simulink model "Demo_FrictionSensor_cs"  (Simulink 7.6)
settings: Solver=ode5  SolverMode=SingleTasking  StartTime=0.0  StopTime=12  FixedStep=1/200  RelTol=1e-3
PreLoadFcn:
  | check_NUTS_defined;
  | 
  | assignin('base',['model_closed_' bdroot],false);
InitFcn:
  | PreScanExperimentInitFcn(bdroot)
StopFcn:
  | PreScanExperimentStopFcn(bdroot)
undefined symbols (not defined in the file): DiscIntNeverNeededParam, warningInitialVelocity, x0, x_ini_VRML, y_ini_VRML, z_ini_VRML
libraries: simulink x40, PreScanSimulinkLibrary x15, simulink_extras x9, PreScanUsefulBlocks x3
(part 4 of 7)

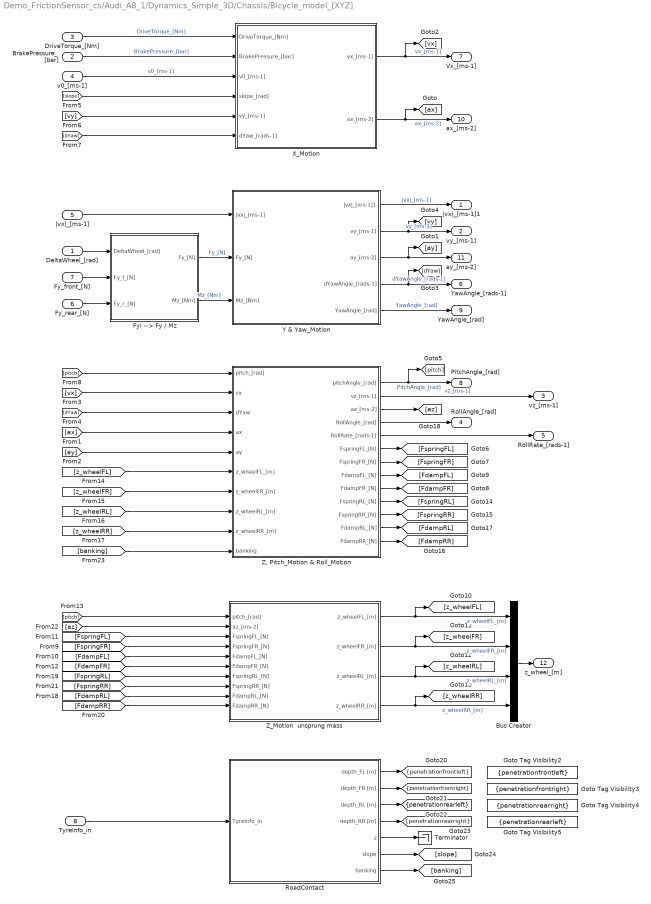
== system Demo_FrictionSensor_cs/Audi_A8_1/Dynamics_Simple_3D/Chassis/Bicycle_model_[XYZ] ==
  DeltaWheel_[rad] : Inport
  BrakePressure_[bar] : Inport  Port=2
  DriveTorque_[Nm] : Inport  Port=3
  v0_[ms-1] : Inport  Port=4
  |vx|_[ms-1] : Inport  Port=5
  Fy_rear_[N] : Inport  Port=6
  Fy_front_[N] : Inport  Port=7
  TyreInfo_in : Inport  Port=8
  Bus Creator : BusCreator
  Fyi --> Fy / Mz : Subsystem
  Goto Tag Visibility2 : GotoTagVisibility  GotoTag=penetrationfrontleft
  Goto Tag Visibility3 : GotoTagVisibility  GotoTag=penetrationfrontright
  Goto Tag Visibility4 : GotoTagVisibility  GotoTag=penetrationrearright
  Goto Tag Visibility5 : GotoTagVisibility  GotoTag=penetrationrearleft
  RoadContact : Subsystem
  Terminator : Terminator
  X_Motion : Subsystem
  Y & Yaw_Motion : Subsystem
  "Z, Pitch_Motion & Roll_Motion" : Subsystem
  Z_Motion  unsprung mass : Subsystem
  |vx|_[ms-1]1 : Outport
  vy_[ms-1] : Outport  Port=2
  vz_[ms-1] : Outport  Port=3
  RollAngle_[rad] : Outport  Port=4
  RollRate_[rads-1] : Outport  Port=5
  YawAngle_[rads-1] : Outport  Port=6
  Vx_[ms-1] : Outport  Port=7
  PitchAngle_[rad] : Outport  Port=8
  YawAngle_[rad] : Outport  Port=9
  ax_[ms-2] : Outport  Port=10
  ay_[ms-2] : Outport  Port=11
  z_wheel_[m] : Outport  Port=12
  tag scope: penetrationfrontleft=scoped, penetrationfrontright=scoped, penetrationrearleft=scoped, penetrationrearright=scoped
  wires:
  [banking] -> "Z, Pitch_Motion & Roll_Motion"/10(banking)
  RoadContact/7(banking) -> [banking]
  RoadContact/6(slope) -> [slope]
  RoadContact/5(z) -> Terminator/1
  "Z, Pitch_Motion & Roll_Motion"/1(pitchAngle_[rad]) -> PitchAngle_[rad]/1, [pitch]  "PitchAngle_[rad]"
  Y & Yaw_Motion/4(dYawAngle_[rads-1]) -> [dYaw], YawAngle_[rads-1]/1  "dYawAngle_[rads-1]"
  [vx] -> "Z, Pitch_Motion & Roll_Motion"/2(vx)
  [dYaw] -> "Z, Pitch_Motion & Roll_Motion"/3(dYaw)
  "Z, Pitch_Motion & Roll_Motion"/4(RollAngle_[rad]) -> RollAngle_[rad]/1
  [ay] -> "Z, Pitch_Motion & Roll_Motion"/5(ay)
  Y & Yaw_Motion/3(ay_[ms-2]) -> ay_[ms-2]/1, [ay]
  |vx|_[ms-1]/1 -> Y & Yaw_Motion/1(|vx|_[ms-1])
  Fy_rear_[N]/1 -> Fyi --> Fy / Mz/3(Fy_r_[N])
  Fy_front_[N]/1 -> Fyi --> Fy / Mz/2(Fy_f_[N])
  DeltaWheel_[rad]/1 -> Fyi --> Fy / Mz/1(DeltaWheel_[rad])
  [ax] -> "Z, Pitch_Motion & Roll_Motion"/4(ax)
  X_Motion/1(vx_[ms-1]) -> [vx], Vx_[ms-1]/1  "vx_[ms-1]"
  X_Motion/2(ax_[ms-2]) -> [ax], ax_[ms-2]/1  "ax_[ms-2]"
  DriveTorque_[Nm]/1 -> X_Motion/1(DriveTorque_[Nm])  "DriveTorque_[Nm]"
  BrakePressure_[bar]/1 -> X_Motion/2(BrakePressure_[bar])  "BrakePressure_[bar]"
  Y & Yaw_Motion/2(vy_[ms-1]) -> vy_[ms-1]/1, [vy]  "vy_[ms-1]"
  Y & Yaw_Motion/1(|vx|_[ms-1]1) -> |vx|_[ms-1]1/1  "|vx|_[ms-1]"
  Fyi --> Fy / Mz/2(Mz_[Nm]) -> Y & Yaw_Motion/3(Mz_[Nm])  "Mz_[Nm]"
  Fyi --> Fy / Mz/1(Fy_[N]) -> Y & Yaw_Motion/2(Fy_[N])  "Fy_[N]"
  [vy] -> X_Motion/5(vy_[ms-1])
  [dYaw] -> X_Motion/6(dYaw_[rads-1])
  "Z, Pitch_Motion & Roll_Motion"/3(az_[ms-2]) -> [az]
  "Z, Pitch_Motion & Roll_Motion"/5(RollRate_[rads-1]) -> RollRate_[rads-1]/1
  "Z, Pitch_Motion & Roll_Motion"/6(FspringFL_[N]) -> [FspringFL]
  "Z, Pitch_Motion & Roll_Motion"/7(FspringFR_[N]) -> [FspringFR]
  "Z, Pitch_Motion & Roll_Motion"/8(FdampFL_[N]) -> [FdampFL]
  "Z, Pitch_Motion & Roll_Motion"/9(FdampFR_[N]) -> [FdampFR]
  "Z, Pitch_Motion & Roll_Motion"/10(FspringRL_[N]) -> [FspringRL]
  "Z, Pitch_Motion & Roll_Motion"/11(FspringRR_[N]) -> [FspringRR]
  "Z, Pitch_Motion & Roll_Motion"/12(FdampRL_[N]) -> [FdampRL]
  "Z, Pitch_Motion & Roll_Motion"/13(FdampRR_[N]) -> [FdampRR]
  [pitch] -> "Z, Pitch_Motion & Roll_Motion"/1(pitch_[rad])
  [z_wheelFL] -> "Z, Pitch_Motion & Roll_Motion"/6(z_wheelFL_[m])
  [z_wheelFR] -> "Z, Pitch_Motion & Roll_Motion"/7(z_wheelFR_[m])
  [z_wheelRL] -> "Z, Pitch_Motion & Roll_Motion"/8(z_wheelRL_[m])
  [z_wheelRR] -> "Z, Pitch_Motion & Roll_Motion"/9(z_wheelRR_[m])
  Z_Motion  unsprung mass/1(z_wheelFL_[m]) -> [z_wheelFL], Bus Creator/1  "z_wheelFL_[m]"
  Z_Motion  unsprung mass/2(z_wheelFR_[m]) -> [z_wheelFR], Bus Creator/2  "z_wheelFR_[m]"
  Z_Motion  unsprung mass/3(z_wheelRL_[m]) -> [z_wheelRL], Bus Creator/3  "z_wheelRL_[m]"
  Z_Motion  unsprung mass/4(z_wheelRR_[m]) -> [z_wheelRR], Bus Creator/4  "z_wheelRR_[m]"
  [pitch] -> Z_Motion  unsprung mass/1(pitch_[rad])
  [FspringFL] -> Z_Motion  unsprung mass/3(FspringFL_[N])
  [FspringFR] -> Z_Motion  unsprung mass/4(FspringFR_[N])
  [FdampFL] -> Z_Motion  unsprung mass/5(FdampFL_[N])
  [FdampFR] -> Z_Motion  unsprung mass/6(FdampFR_[N])
  [FspringRL] -> Z_Motion  unsprung mass/7(FspringRL_[N])
  [FspringRR] -> Z_Motion  unsprung mass/8(FspringRR_[N])
  [FdampRL] -> Z_Motion  unsprung mass/9(FdampRL_[N])
  [FdampRR] -> Z_Motion  unsprung mass/10(FdampRR_[N])
  [az] -> Z_Motion  unsprung mass/2(az_[ms-2])
  Y & Yaw_Motion/5(YawAngle_[rad]) -> YawAngle_[rad]/1  "YawAngle_[rad]"
  RoadContact/1(depth_FL [m]) -> [penetrationfrontleft]
  RoadContact/2(depth_FR [m]) -> [penetrationfrontright]
  RoadContact/3(depth_RL [m]) -> [penetrationrearleft]
  RoadContact/4(depth_RR [m]) -> [penetrationrearright]
  [slope] -> X_Motion/4(slope_[rad])
  v0_[ms-1]/1 -> X_Motion/3(v0_[ms-1])  "v0_[ms-1]"
  "Z, Pitch_Motion & Roll_Motion"/2(vz_[ms-1]) -> vz_[ms-1]/1  "vz_[ms-1]"
  Bus Creator/1 -> z_wheel_[m]/1
  TyreInfo_in/1 -> RoadContact/1(TyreInfo_in)

== system Demo_FrictionSensor_cs/Audi_A8_1/Dynamics_Simple_3D/Chassis/FrontTyre ==
  note: alpha limiter
      | [-1 ... 1]
  note: VEHICLE + MOTORCYCLE
  note: MOTORCYCLE ONLY
  note: relax_on
      | ON: 1
      | OFF: 0
  DeltaWheel_[rad] : Inport
  |vx|_[ms-1] : Inport  Port=2
  vy_[ms-1] : Inport  Port=3
  dYawAngle_[rads-1] : Inport  Port=4
  RollAngle_[rad] : Inport  Port=5
  AlphaFront : Subsystem
  Compare To Zero : simulink/Logic and Bit Operations/Compare To Zero  SystemSampleTime=-1  relop===  LogicOutDataTypeMode=boolean  ZeroCross=off
  Configurable Subsystem : Subsystem  BlockChoice=Discrete-Time Integrator  mask{ComputationMode=ComputationMode}
      mask prompts: ComputationMode "Computation mode:"
      mask init:
      | SetComputationMode(gcb,ComputationMode);
      settings: AttributesFormatString=%<BlockChoice>  OpenFcn=BringToFront(gcb);  MemberBlocks=Discrete-Time Integrator,Integrator
      settings: TemplateBlock=|
      | PreScanSimulinkLibrary/Configurable Subsystems/integral with reset and limits
      | for slip angle/Configurable
      | Subsystem
  Configurable Subsystem1 : Subsystem  BlockChoice=Discrete-Time Integrator  mask{ComputationMode=ComputationMode}
      mask prompts: ComputationMode "Computation mode:"
      mask init:
      | SetComputationMode(gcb,ComputationMode);
      settings: AttributesFormatString=%<BlockChoice>  OpenFcn=BringToFront(gcb);  MemberBlocks=Discrete-Time Integrator,Integrator
      settings: TemplateBlock=|
      | PreScanSimulinkLibrary/Configurable Subsystems/integral with reset/Configurable
      | Subsystem
  Constant : Constant  Value=p.relax_on
  Constant1 : Constant  Value=p.relax_on
  Constant2 : Constant  Value=p.VehMCSwitch
  Data Type Conversion : DataTypeConversion  OutDataTypeStr=double
  If MC : simulink/Logic and Bit Operations/Compare To Constant  SystemSampleTime=-1  relop===  const=2  LogicOutDataTypeMode=uint8  ZeroCross=off
  K_gamma_front : Gain  Gain=p.Kgfront
  Linl : Fcn  Expr=(u(4) - u(5))/p.sigma_front*u(1)
  Linl1 : Fcn  Expr=(u(4) - u(5))/p.sigma_front*u(1)
  Mux1 : Mux  Inputs=3
  Mux2 : Mux  Inputs={3,1,1}
  Mux3 : Mux  Inputs={3,1,1}
  Product : Product  RndMeth=Zero
  Sum : Sum  Inputs=|++  SaturateOnIntegerOverflow=on  InputSameDT=on  OutDataTypeStr=Inherit: Same as first input
  Sum1 : Sum  Inputs=|++
  Switch : Switch  Threshold=0.5  SaturateOnIntegerOverflow=on  InputSameDT=on
  Switch1 : Switch  Threshold=0.5  SaturateOnIntegerOverflow=on  InputSameDT=on
  alg.loop : Memory
  due to sign convention : Gain  Gain=-1  SaturateOnIntegerOverflow=on  OutDataTypeStr=Inherit: Same as input  ParamDataTypeStr=Inherit: Same as input
  front_tyre : Gain  Gain=p.Kfront
  FyFront_[N] : Outport
  wires:
  Switch1/1 -> K_gamma_front/1  "GammaFront_[rad]"
  DeltaWheel_[rad]/1 -> Sum/2  "DeltaWheel_[rad]"
  [reset] -> Configurable Subsystem1/2(In2)
  [reset] -> Configurable Subsystem/2(In2)
  Compare To Zero/1 -> [reset]
  Data Type Conversion/1 -> Product/2
  Product/1 -> Sum1/2
  K_gamma_front/1 -> Product/1
  If MC/1 -> Data Type Conversion/1
  Constant2/1 -> If MC/1
  front_tyre/1 -> Sum1/1
  RollAngle_[rad]/1 -> due to sign convention/1
  due to sign convention/1 -> Mux3/2, alg.loop/1  "GammaStatFront_[rad]"
  Constant1/1 -> Switch1/2
  Mux3/1 -> Linl1/1
  Linl1/1 -> Configurable Subsystem1/1(In1)
  Configurable Subsystem1/1(Out1) -> Switch1/1, Mux3/3  "GammaRelaxFront_[rad]"
  alg.loop/1 -> Switch1/3
  dYawAngle_[rads-1]/1 -> Mux1/3
  vy_[ms-1]/1 -> Mux1/2
  |vx|_[ms-1]/1 -> Compare To Zero/1, Mux1/1
  Mux1/1 -> Mux3/1, Mux2/1, AlphaFront/1(In)
  AlphaFront/1(Alpha) -> Sum/1
  Configurable Subsystem/1(Out1) -> Switch/1, Mux2/3  "AlphaRelaxFront_[rad]"
  Linl/1 -> Configurable Subsystem/1(In1)
  Mux2/1 -> Linl/1
  Sum1/1 -> FyFront_[N]/1  "FyFront_[N]"
  Constant/1 -> Switch/2
  Switch/1 -> front_tyre/1  "AlphaFront_[rad]"
  Sum/1 -> Switch/3, Mux2/2  "AlphaStatFront_[rad]"

== system Demo_FrictionSensor_cs/Audi_A8_1/Dynamics_Simple_3D/Chassis/Power Assisted Steering ==
  note: Reverse steering direction for negative velocities
  note: VEHICLE
  note: MOTORCYCLE
  Vx_[ms-1] : Inport
  Delta_in_[deg] : Inport  Port=2
  Constant : Constant
  Constant1 : Constant  Value=p.VehMCSwitch
  Lookup Table : Lookup  InputValues=[0 35 45 100]  Table=[1 1 0.2 0.2]
  Multiport Switch : MultiPortSwitch  Inputs=2  zeroidx=off
  Product : Product  Inputs=3  RndMeth=Zero
  Sign : Signum
  Delta_out_[deg] : Outport
  wires:
  Sign/1 -> Product/1
  Product/1 -> Delta_out_[deg]/1
  Multiport Switch/1 -> Product/2
  Lookup Table/1 -> Multiport Switch/2
  Constant/1 -> Multiport Switch/3
  Constant1/1 -> Multiport Switch/1
  Delta_in_[deg]/1 -> Product/3
  Vx_[ms-1]/1 -> Sign/1, Lookup Table/1

== system Demo_FrictionSensor_cs/Audi_A8_1/Dynamics_Simple_3D/Chassis/RearTyre ==
  note: alpha limiter
      | [-1 ... 1]
  note: VEHICLE + MOTORCYCLE
  note: MOTORCYCLE ONLY
  note: relax_on
      | ON: 1
      | OFF: 0
  |vx|_[ms-1] : Inport
  vy_[ms-1] : Inport  Port=2
  dpsi_[rads-1] : Inport  Port=3
  RollAngle_[rad] : Inport  Port=4
  AlphaRear : Subsystem
  Compare To Zero : simulink/Logic and Bit Operations/Compare To Zero  SystemSampleTime=-1  relop===  LogicOutDataTypeMode=boolean  ZeroCross=off
  Configurable Subsystem : Subsystem  BlockChoice=Discrete-Time Integrator  mask{ComputationMode=ComputationMode}
      mask prompts: ComputationMode "Computation mode:"
      mask init:
      | SetComputationMode(gcb,ComputationMode);
      settings: AttributesFormatString=%<BlockChoice>  OpenFcn=BringToFront(gcb);  MemberBlocks=Discrete-Time Integrator,Integrator
      settings: TemplateBlock=|
      | PreScanSimulinkLibrary/Configurable Subsystems/integral with reset and limits
      | for slip angle/Configurable
      | Subsystem
  Configurable Subsystem1 : Subsystem  BlockChoice=Discrete-Time Integrator  mask{ComputationMode=ComputationMode}
      mask prompts: ComputationMode "Computation mode:"
      mask init:
      | SetComputationMode(gcb,ComputationMode);
      settings: AttributesFormatString=%<BlockChoice>  OpenFcn=BringToFront(gcb);  MemberBlocks=Discrete-Time Integrator,Integrator
      settings: TemplateBlock=|
      | PreScanSimulinkLibrary/Configurable Subsystems/integral with reset/Configurable
      | Subsystem
  Constant1 : Constant  Value=p.relax_on
  Constant2 : Constant  Value=p.relax_on
  Constant3 : Constant  Value=p.VehMCSwitch
  Data Type Conversion : DataTypeConversion  OutDataTypeStr=double
  If MC : simulink/Logic and Bit Operations/Compare To Constant  SystemSampleTime=-1  relop===  const=2  LogicOutDataTypeMode=uint8  ZeroCross=off
  K_gamma_rear : Gain  Gain=p.Kgrear
  Linl : Fcn  Expr=(u(4) - u(5))/p.sigma_rear*u(1)
  Linl1 : Fcn  Expr=(u(4) - u(5))/p.sigma_rear*u(1)
  Mux1 : Mux  Inputs=3
  Mux2 : Mux  Inputs={3,1,1}
  Mux3 : Mux  Inputs={3,1,1}
  Product : Product  RndMeth=Zero
  Sum1 : Sum  Inputs=|++
  Switch1 : Switch  Threshold=0.5  SaturateOnIntegerOverflow=on  InputSameDT=on
  Switch2 : Switch  Threshold=0.5  SaturateOnIntegerOverflow=on  InputSameDT=on
  alg.loop : Memory
  due to sign convention : Gain  Gain=-1  SaturateOnIntegerOverflow=on  OutDataTypeStr=Inherit: Same as input  ParamDataTypeStr=Inherit: Same as input
  rear_tyre : Gain  Gain=p.Krear
  FyRear_[N] : Outport
  wires:
  Switch2/1 -> K_gamma_rear/1  "GammaFront_[rad]"
  [reset] -> Configurable Subsystem1/2(In2)
  [reset] -> Configurable Subsystem/2(In2)
  Compare To Zero/1 -> [reset]
  rear_tyre/1 -> Sum1/1
  K_gamma_rear/1 -> Product/1
  Data Type Conversion/1 -> Product/2
  Product/1 -> Sum1/2
  If MC/1 -> Data Type Conversion/1
  Constant3/1 -> If MC/1
  RollAngle_[rad]/1 -> due to sign convention/1
  due to sign convention/1 -> Mux3/2, alg.loop/1  "GammaStatRear_[rad]"
  Constant2/1 -> Switch2/2
  Mux3/1 -> Linl1/1
  Linl1/1 -> Configurable Subsystem1/1(In1)
  Configurable Subsystem1/1(Out1) -> Switch2/1, Mux3/3  "GammaRelaxRear_[rad]"
  alg.loop/1 -> Switch2/3
  dpsi_[rads-1]/1 -> Mux1/3
  vy_[ms-1]/1 -> Mux1/2
  |vx|_[ms-1]/1 -> Compare To Zero/1, Mux1/1
  Mux1/1 -> Mux3/1, Mux2/1, AlphaRear/1(In)
  Configurable Subsystem/1(Out1) -> Switch1/1, Mux2/3  "AlphaRelaxRear_[rad]"
  Linl/1 -> Configurable Subsystem/1(In1)
  Mux2/1 -> Linl/1
  Sum1/1 -> FyRear_[N]/1  "FyRear_[N]"
  Constant1/1 -> Switch1/2
  Switch1/1 -> rear_tyre/1  "AlphaRear_[rad]"
  AlphaRear/1(Alpha) -> Mux2/2, Switch1/3  "AlphaStatRear_[rad]"

== system Demo_FrictionSensor_cs/Audi_A8_1/Dynamics_Simple_3D/Engine/Configurable Subsystem ==
  In1 : Inport
  Discrete Rate Limiter : DiscreteTransferFcn  Numerator="[  1-exp(-( (TimeStep) / 0.1) )  ]"  Denominator="[  1   -exp(-( (TimeStep) / 0.1) )   ]"  SampleTime=TimeStep
  Out1 : Outport
  wires:
  Discrete Rate Limiter/1 -> Out1/1
  In1/1 -> Discrete Rate Limiter/1

== system Demo_FrictionSensor_cs/Audi_A8_1/Dynamics_Simple_3D/Engine/Configurable Subsystem1 ==
  In1 : Inport
  Discrete-Time Integrator : DiscreteIntegrator  InitialCondition=p.rot_ini  SampleTime=TimeStep  LimitOutput=on  UpperSaturationLimit=p.rot_upp  LowerSaturationLimit=p.rot_low  ICPrevOutput=DiscIntNeverNeededParam  ICPrevScaledInput=DiscIntNeverNeededParam
  Out1 : Outport
  wires:
  Discrete-Time Integrator/1 -> Out1/1
  In1/1 -> Discrete-Time Integrator/1

== system Demo_FrictionSensor_cs/Audi_A8_1/Dynamics_Simple_3D/Gear: Auto Manual/If Action Subsystem ==
  In1 : Inport
  Action Port : ActionPort  PropagateVarSize=During execution
  Out1 : Outport
  wires:
  In1/1 -> Out1/1

== system Demo_FrictionSensor_cs/Audi_A8_1/Dynamics_Simple_3D/Gear: Auto Manual/If Action Subsystem1 ==
  In1 : Inport
  Action Port : ActionPort  PropagateVarSize=During execution
  Out1 : Outport
  wires:
  In1/1 -> Out1/1

== system Demo_FrictionSensor_cs/Audi_A8_1/Dynamics_Simple_3D/ShiftLogic/Detect Increase ==
  GearNr_[-] : Inport
  In2 : Inport  Port=2
  Constant : Constant
  Data Type Conversion : DataTypeConversion  OutDataTypeStr=double
  Data Type Conversion1 : DataTypeConversion  OutDataTypeStr=double
  Detect Increase : simulink/Logic and Bit Operations/Detect Increase  SystemSampleTime=-1  vinit=1
  If : If  NumInputs=2  IfExpression="u1==1 &  u2==1"
  If V0 higher of the from 2->3 shifting velocity : Subsystem  TreatAsAtomicUnit=on
  Merge : Merge
  Other : Subsystem  TreatAsAtomicUnit=on
  Out1 : Outport
  wires:
  If/2 -> Other/Action
  If V0 higher of the from 2->3 shifting velocity/1(Out1) -> Merge/1
  Other/1(Out1) -> Merge/2
  Detect Increase/1 -> Data Type Conversion/1
  Merge/1 -> Out1/1
  If/1 -> If V0 higher of the from 2->3 shifting velocity/Action
  Data Type Conversion1/1 -> If/2
  Data Type Conversion/1 -> If/1
  Constant/1 -> If V0 higher of the from 2->3 shifting velocity/1(In1)
  GearNr_[-]/1 -> Detect Increase/1
  In2/1 -> Data Type Conversion1/1, Other/1(In1)

== system Demo_FrictionSensor_cs/Audi_A8_1/Dynamics_Simple_3D/ShiftLogic/If Action Neutral ==
  In1 : Inport
  Action Port : ActionPort  InitializeStates=reset  PropagateVarSize=During execution
  Out1 : Outport
  wires:
  In1/1 -> Out1/1

== system Demo_FrictionSensor_cs/Audi_A8_1/Dynamics_Simple_3D/ShiftLogic/If Action Normal ==
  In1 : Inport
  Action Port : ActionPort  InitializeStates=reset  PropagateVarSize=During execution
  Out1 : Outport
  wires:
  In1/1 -> Out1/1

== system Demo_FrictionSensor_cs/Audi_A8_1/Dynamics_Simple_3D/ShiftLogic/If Action Reverse ==
  In1 : Inport
  Action Port : ActionPort  InitializeStates=reset  PropagateVarSize=During execution
  Out1 : Outport
  wires:
  In1/1 -> Out1/1

== system Demo_FrictionSensor_cs/Audi_A8_1/Dynamics_Simple_3D/Transmission/Torque_Converter ==
  note: To compensate for no hydraulic connection when in neutral gear
  note: > 0
  note: <= 0
  nEngine_[rpm] : Inport
  nTransmission_[rpm] : Inport  Port=2
  Gear nr : Inport  Port=3
  Compare To Constant : simulink/Logic and Bit Operations/Compare To Constant  SystemSampleTime=-1  relop=<=  const=1  LogicOutDataTypeMode=uint8  ZeroCross=off
  Compare To Zero : simulink/Logic and Bit Operations/Compare To Zero  SystemSampleTime=-1  relop=~=  LogicOutDataTypeMode=uint8  ZeroCross=off
  Constant : Constant  Value=1/50
  Constant1 : Constant
  Constant2 : Constant
  Drag : Gain  Gain=-1
  FactorK : Lookup  InputValues=p.speedratio  Table=p.Kfactor*p.Kcorr  SaturateOnIntegerOverflow=on
  Impeller : Fcn  Expr=u^2
  Product : Product  RndMeth=Zero
  Product1 : Product  RndMeth=Zero
  Quotient : Product  Inputs=*/  SaturateOnIntegerOverflow=on  InputSameDT=on  OutDataTypeStr=Inherit: Same as first input
  SpeedRatio : Product  Inputs=*/  SaturateOnIntegerOverflow=on  InputSameDT=on  OutDataTypeStr=Inherit: Same as first input
  Sum : Sum  Inputs=|+-
  Switch : Switch  Criteria=u2 ~= 0  Threshold=0.5
  Switch1 : Switch  Criteria=u2 ~= 0
  TorqueRatio : Lookup  InputValues=[p.speedratio 1]  Table=[p.Torqueratio 0]  SaturateOnIntegerOverflow=on
  Turbine : Product  SaturateOnIntegerOverflow=on  InputSameDT=on  OutDataTypeStr=Inherit: Same as first input
  ImpellerTorque_[Nm] : Outport  InitialOutput=0
  TurbineTorque_[Nm] : Outport  Port=2  InitialOutput=0
  wires:
  nTransmission_[rpm]/1 -> SpeedRatio/1
  nEngine_[rpm]/1 -> Quotient/1, SpeedRatio/2
  Impeller/1 -> Product/2, Turbine/1
  SpeedRatio/1 -> FactorK/1, TorqueRatio/1, Compare To Constant/1, Sum/1
  FactorK/1 -> Quotient/2
  Quotient/1 -> Impeller/1
  Product/1 -> ImpellerTorque_[Nm]/1
  Switch/1 -> Product/1, Product1/1
  Constant/1 -> Switch/3
  Constant1/1 -> Switch/1
  Gear nr/1 -> Compare To Zero/1
  Compare To Zero/1 -> Switch/2
  Switch1/1 -> Product1/2
  Product1/1 -> TurbineTorque_[Nm]/1
  Drag/1 -> Switch1/3
  Sum/1 -> Drag/1
  Constant2/1 -> Sum/2
  Compare To Constant/1 -> Switch1/2
  TorqueRatio/1 -> Turbine/2
  Turbine/1 -> Switch1/1

== system Demo_FrictionSensor_cs/Audi_A8_1/Dynamics_Simple_3D/Transmission/Transmission_Ratio ==
  tTransmissionIn_[Nm] : Inport
  GearNr_[-] : Inport  Port=2
  nTransmissionOut_[rpm] : Inport  Port=3
  Ensure positive TransmissionRPM : Abs
  If : If  IfExpression=u1 == 0  ElseIfExpressions=u1 == -1
  If Action Neutral : Subsystem  TreatAsAtomicUnit=on
  If Action Normal : Subsystem  TreatAsAtomicUnit=on
  If Action Reverse : Subsystem  TreatAsAtomicUnit=on
  Merge : Merge  Inputs=3
  OutputTorque = 0 : Constant  Value=0
  Product : Product  SaturateOnIntegerOverflow=on  InputSameDT=on  OutDataTypeStr=Inherit: Same as first input
  Product1 : Product  SaturateOnIntegerOverflow=on  InputSameDT=on  OutDataTypeStr=Inherit: Same as first input
  Transmission Gear ratios : Lookup  InputValues=p.tr_in  Table=p.tr_out  SaturateOnIntegerOverflow=on
  tTransmissionOut_[Nm] : Outport  InitialOutput=0
  nTransmissionIn_[rpm] : Outport  Port=2  InitialOutput=0
  wires:
  GearNr_[-]/1 -> Transmission Gear ratios/1, If/1
  If/3 -> If Action Normal/Action
  If/2 -> If Action Reverse/Action
  If Action Normal/1(Out1) -> Merge/3
  If Action Reverse/1(Out1) -> Merge/2
  If/1 -> If Action Neutral/Action
  If Action Neutral/1(Out1) -> Merge/1
  Product1/1 -> Ensure positive TransmissionRPM/1
  Merge/1 -> tTransmissionOut_[Nm]/1
  Product/1 -> If Action Reverse/1(In1), If Action Normal/1(In1)
  OutputTorque = 0/1 -> If Action Neutral/1(In1)
  Transmission Gear ratios/1 -> Product/2, Product1/1
  nTransmissionOut_[rpm]/1 -> Product1/2
  tTransmissionIn_[Nm]/1 -> Product/1
  Ensure positive TransmissionRPM/1 -> nTransmissionIn_[rpm]/1

== system Demo_FrictionSensor_cs/Audi_A8_1/PathFollower_Preview_1/LateralController/CTRL REFERENCES ==
  note: REFERENCE POSITION BASED POSITION CTRL
  Pos x,y,Y [m,m,rad] : Inport
  Position Preview Distance [m] : Inport  Port=2
  TrajOffset [m,m,rad] : Inport  Port=3
  ActorOffset_Left(+) / Right(-)_[m] : Inport  Port=4
  Calculate Lateral Error : Subsystem
      mask Display:
      | port_label('input',1,'pvp');
      | port_label('input',2,'TrajOffset_x_y_Y');
      | port_label('input',3,'ActorOffset_Left_Right');
      | port_label('input',4,'p0');
      | port_label('input',5,'PreviewDistance');
      | port_label('output',1,'dist_psvehicle');
  Calculate Preview Point (pvp) by extrapolating current Vehicle Position (p0) with Preview Distance and Vehicle Orientation : Subsystem
  Find Reference Point (pref0) on Trajectory closest to P0 Point (p0) : Subsystem
      mask Display:
      | port_label('input',1,'pvp');
      | port_label('input',2,'TrajOffset_x_y_Y');
      | port_label('input',3,'ActorOffset_Left_Right');
      | port_label('input',4,'p0');
      | port_label('output',1,'Actor_traj_distance');
      | port_label('output',2,'Actor_traj_angle');
  Mux1 : Mux  Inputs=2
  Selector2 : Selector  InputPortWidth=3  IndexOptions=Index vector (dialog)  Indices=[1 2]  OutputSizes=1
  Terminator : Terminator
  Actor/Traj_distance [m] : Outport
  Actor/Traj_angle [deg] : Outport  Port=2
  e_Lat [m] : Outport  Port=3
  wires:
  Mux1/1 -> Calculate Lateral Error/1(In1), Find Reference Point (pref0) on Trajectory closest to P0 Point (p0)/1(In1)
  Pos x,y,Y [m,m,rad]/1 -> Calculate Preview Point (pvp) by extrapolating current Vehicle Position (p0) with Preview Distance and Vehicle Orientation/2(x,y,Y Demux [m,m,rad]), Find Reference Point (pref0) on Trajectory closest to P0 Point (p0)/4(In4), Selector2/1
  Calculate Preview Point (pvp) by extrapolating current Vehicle Position (p0) with Preview Distance and Vehicle Orientation/1(x_glob_PVP) -> Mux1/1
  Position Preview Distance [m]/1 -> Calculate Lateral Error/5(In5), Calculate Preview Point (pvp) by extrapolating current Vehicle Position (p0) with Preview Distance and Vehicle Orientation/1(Preview Distance)
  Calculate Preview Point (pvp) by extrapolating current Vehicle Position (p0) with Preview Distance and Vehicle Orientation/2(y_glob_PVP) -> Mux1/2
  TrajOffset [m,m,rad]/1 -> Find Reference Point (pref0) on Trajectory closest to P0 Point (p0)/2(In2), Calculate Lateral Error/2(In2)  "L6"
  ActorOffset_Left(+) / Right(-)_[m]/1 -> Find Reference Point (pref0) on Trajectory closest to P0 Point (p0)/3(In3), Calculate Lateral Error/3(In3)
  Find Reference Point (pref0) on Trajectory closest to P0 Point (p0)/1(Out1) -> Actor/Traj_distance [m]/1
  Find Reference Point (pref0) on Trajectory closest to P0 Point (p0)/2(Out2) -> Actor/Traj_angle [deg]/1
  Calculate Preview Point (pvp) by extrapolating current Vehicle Position (p0) with Preview Distance and Vehicle Orientation/3(Y [rad]) -> Terminator/1
  Calculate Lateral Error/1(Out1) -> e_Lat [m]/1
  Selector2/1 -> Calculate Lateral Error/4(In4)

== system Demo_FrictionSensor_cs/Audi_A8_1/PathFollower_Preview_1/LateralController/Calculate delta steering error ==
  In1 : Inport
  In2 : Inport  Port=2
  In3 : Inport  Port=3
  In4 : Inport  Port=4
  In5 : Inport  Port=5
  In6 : Inport  Port=6
  In7 : Inport  Port=7
  In8 : Inport  Port=8
  In9 : Inport  Port=9
  In10 : Inport  Port=10
  In11 : Inport  Port=11
  In12 : Inport  Port=12
  eml_delta_steering_error : Stateflow chart  TreatAsAtomicUnit=on  RTWFcnName=sfun_delta_steering_error  RTWFileName=sfun_delta_steering_error
      settings: RTWFcnNameOpts=User specified  RTWFileNameOpts=User specified
  Out1 : Outport
  wires:
  In3/1 -> eml_delta_steering_error/3(t_Preview_LatCtrl)
  In2/1 -> eml_delta_steering_error/2(v_x_vehicle_Min)
  In12/1 -> eml_delta_steering_error/12(wheelbase)
  In11/1 -> eml_delta_steering_error/11(Pos_x_CoG_Vehicle)
  In10/1 -> eml_delta_steering_error/10(e_Lat)
  In9/1 -> eml_delta_steering_error/9(inertia_z_vehicle_total)
  In8/1 -> eml_delta_steering_error/8(m_vehicle_total)
  eml_delta_steering_error/1(delta_steeringwheeltotal) -> Out1/1
  In7/1 -> eml_delta_steering_error/7(CorneringStiffness_Tyres_Rear)
  In6/1 -> eml_delta_steering_error/6(CorneringStiffness_Tyres_Front)
  In5/1 -> eml_delta_steering_error/5(yawrate_vehicle)
  In4/1 -> eml_delta_steering_error/4(v_y_vehicle)
  In1/1 -> eml_delta_steering_error/1(v_x_vehicle)

== system Demo_FrictionSensor_cs/Audi_A8_1/PathFollower_Preview_1/LateralController/SteeringWheelAngle ==
  Angle_Steering[rad] : Inport
  i_Steering[] : Inport  Port=2
  Angle_SteeringWheel_Last[deg] : Inport  Port=3
  LatCtrl1_Enable[0Off|1On] : Inport  Port=4
  Angle_Max_SteeringWheel[deg]1 : Constant  Value=Angle_Max_SteeringWheel  SampleTime=CSSampleTime
  Const_t_PT1_LatCtrl[s] : Constant  Value=DelayTime  SampleTime=CSSampleTime
  FirstOrderDynamics : Subsystem
      mask Type: First Order Dynamics
      mask Display:
      | port_label('input',1,'In')
      | port_label('input',2,'T')
      | port_label('input',3,'Reset')
      | port_label('input',4,'x0')
      | 
      | plot([0.4 0.95], [0.1 0.1]);
      | plot([0.4 0.4], [0.1 0.95]);
      | plot(0.4 + 0.5*[0:0.1:1],0.8- 0.7 * exp(-5*[0:0.1:1]));
  Gain : Gain  SaturateOnIntegerOverflow=on  OutDataTypeStr=Inherit: Same as input  ParamDataTypeStr=Inherit: Same as input
  Product : Product  SaturateOnIntegerOverflow=on  OutDataTypeStr=Inherit: Same as first input
  Rate Limiter : RateLimiter  RisingSlewLimit=MaxSteeringRate  FallingSlewLimit=-MaxSteeringRate  SampleTimeMode=inherited
  Sat_Total : Subsystem
      mask Display:
      | plot([0.25 0.4 0.6 0.75],[0.2 0.2 0.8 0.8])
      | port_label('input',2,'Lim')
      | port_label('output',2,'Info')
  Terminator1 : Terminator
  rad2deg : Gain  Gain=180/pi  SaturateOnIntegerOverflow=on  OutDataTypeStr=Inherit: Same as input  ParamDataTypeStr=Inherit: Same as input
  Angle_SteeringWheel[deg] : Outport
  wires:
  Rate Limiter/1 -> FirstOrderDynamics/1(In)
  Gain/1 -> FirstOrderDynamics/3(Reset)
  Angle_SteeringWheel_Last[deg]/1 -> FirstOrderDynamics/4(x0)
  LatCtrl1_Enable[0Off|1On]/1 -> Gain/1
  Const_t_PT1_LatCtrl[s]/1 -> FirstOrderDynamics/2(TimeConstant[s])
  Sat_Total/2(Sat_Info) -> Terminator1/1
  Angle_Steering[rad]/1 -> rad2deg/1
  i_Steering[]/1 -> Product/2
  rad2deg/1 -> Product/1
  Product/1 -> Sat_Total/1(In)
  Sat_Total/1(Sat_Total) -> Rate Limiter/1
  FirstOrderDynamics/1(Out) -> Angle_SteeringWheel[deg]/1
  Angle_Max_SteeringWheel[deg]1/1 -> Sat_Total/2(Sat_Limit)

== system Demo_FrictionSensor_cs/Audi_A8_1/PathFollower_Preview_1/LateralController/s_Preview_LatCtrl ==
  v_x_Vehicle[m|s] : Inport
  v_x_Vehicle_Min[m|s] : Inport  Port=2
  t_Preview_LatCtrl[s] : Inport  Port=3
  Const_s_Preview_LatCtrl_Spacing[0_1] : Constant  Value=[0.1, 0.2, 0.3, 0.4, 0.5, 0.6, 0.7, 0.8,0.9, 1.0]  SampleTime=CSSampleTime
  Max : MinMax  Function=max  Inputs=2  SaturateOnIntegerOverflow=on  InputSameDT=on
  Prod_s_Min : Product  SaturateOnIntegerOverflow=on  OutDataTypeStr=Inherit: Same as first input
  Product : Product  SaturateOnIntegerOverflow=on  OutDataTypeStr=Inherit: Same as first input
  Product1 : Product  SaturateOnIntegerOverflow=on  OutDataTypeStr=Inherit: Same as first input
  s_Preview_LatCtrl[m] : Outport
  wires:
  Prod_s_Min/1 -> Max/2
  v_x_Vehicle_Min[m|s]/1 -> Prod_s_Min/2
  t_Preview_LatCtrl[s]/1 -> Prod_s_Min/1, Product/2
  Const_s_Preview_LatCtrl_Spacing[0_1]/1 -> Product1/2
  Max/1 -> Product1/1
  Product/1 -> Max/1
  v_x_Vehicle[m|s]/1 -> Product/1
  Product1/1 -> s_Preview_LatCtrl[m]/1

== system Demo_FrictionSensor_cs/Audi_A8_1/PathFollower_Preview_1/LongitudinalController/Check_Initial_Velocity ==
  " v_actual_[m|s]" : Inport
  Initial_Velocity_[m|s] : Inport  Port=2
  > eps : simulink/Logic and Bit Operations/Compare To Constant  SystemSampleTime=-1  relop=>  const=0.1  LogicOutDataTypeMode=boolean
  Abs : Abs
  Assertion : Assertion  Enabled=on  AssertionFailFcn=warningInitialVelocity(blockPath);  StopWhenAssertionFail=off
  Constant : Constant  Value=false
  First ? : Memory  X0=1
  Logical Operator : Logic  AllPortsSameDT=off  OutDataTypeStr=boolean
  Logical Operator1 : Logic  Operator=NOT  AllPortsSameDT=off  OutDataTypeStr=boolean
  Sum : Sum  Inputs=+-
  wires:
  Logical Operator1/1 -> Assertion/1
  Logical Operator/1 -> Logical Operator1/1
  Constant/1 -> First ?/1
  First ?/1 -> Logical Operator/2
  > eps/1 -> Logical Operator/1
  Sum/1 -> Abs/1
  Abs/1 -> > eps/1
  Initial_Velocity_[m|s]/1 -> Sum/2
  " v_actual_[m|s]"/1 -> Sum/1

== system Demo_FrictionSensor_cs/Audi_A8_1/PathFollower_Preview_1/LongitudinalController/If Desired Velocity = 0 ==
  In1 : Inport
  Action Port : ActionPort  InitializeStates=reset  PropagateVarSize=During execution
  constant : Constant  Value=0
  constant1 : Constant  Value=150
  throttle [%] : Outport  InitialOutput=[0]
  brake pressure [bar] : Outport  Port=2  InitialOutput=[150]
  Auto_GearShift : Outport  Port=3
  wires:
  In1/1 -> Auto_GearShift/1
  constant/1 -> throttle [%]/1
  constant1/1 -> brake pressure [bar]/1

== system Demo_FrictionSensor_cs/Audi_A8_1/PathFollower_Preview_1/LongitudinalController/If Desired Velocity ~= 0 ==
  note: No brake/throttle actions
      | in case of small ctrl error,
      |  in order to prevent nervous
      | ctrl behaviour
  note: CONSTANT VELOCITY CONTROL
  In1 : Inport
  Desired Velocity [m/s] : Inport  Port=2
  Action Port : ActionPort  InitializeStates=reset  PropagateVarSize=During execution
  Dead Zone : DeadZone  LowerValue=-10  UpperValue=1  SaturateOnIntegerOverflow=on
  Gain11 : Gain  Gain=10
  Gain6 : Gain  Gain=-1
  Limiter_brake : Saturate  UpperLimit=150  LowerLimit=0
  Limiter_throttle : Saturate  UpperLimit=100  LowerLimit=0
  PID Controller : Subsystem  mask(PID Controller){P=20, I=0.3, D=3.065}
      mask prompts: P "Proportional:"; I "Integral:"; D "Derivative:"
      mask help:
      | Enter expressions for proportional, integral, and derivative terms.
      | P+I/s+Ds
      mask Help: This block implements a PID controller where parameters are entered for the Proportional, Integral and Derivative terms. Unmask this block to see how it works. The derivative term is implemented using a true derivative block.
      mask Display: disp('PID')
  throttle [%] : Outport
  brake pressure [bar] : Outport  Port=2
  Auto_GearShift : Outport  Port=3
  wires:
  In1/1 -> Auto_GearShift/1
  PID Controller/1(u) -> Dead Zone/1
  Desired Velocity [m/s]/1 -> PID Controller/1(e)
  Dead Zone/1 -> Gain11/1, Limiter_throttle/1
  Gain11/1 -> Gain6/1
  Gain6/1 -> Limiter_brake/1
  Limiter_brake/1 -> brake pressure [bar]/1
  Limiter_throttle/1 -> throttle [%]/1  "throttle"

== system Demo_FrictionSensor_cs/Audi_A8_1/PathFollower_Preview_1/LongitudinalController/Memory External IC ==
  note: Xnew
  note: Initial Value
  u : Inport
  IC : Inport  Port=2
  FixPt Constant : Constant  DisableCoverage=on  Value=0  OutDataTypeStr=fixdt(0,8,0)
  FixPt Data Type Duplicate1 : DataTypeDuplicate  DisableCoverage=on  NumInputPorts=3
  Init : Switch  Criteria=u2 ~= 0  OutDataTypeStr=Inherit: Inherit via back propagation  ZeroCross=off
  Memory : Memory  X0=1  InheritSampleTime=on
  Memory1 : Memory  InheritSampleTime=on
  y : Outport
  wires:
  Memory1/1 -> Init/3  "Xold"
  Init/1 -> y/1, FixPt Data Type Duplicate1/1
  Memory/1 -> Init/2
  FixPt Constant/1 -> Memory/1
  u/1 -> Memory1/1, FixPt Data Type Duplicate1/2
  IC/1 -> Init/1, FixPt Data Type Duplicate1/3

== system Demo_FrictionSensor_cs/Audi_A8_1/PreScan_Contact_Sensor/Tire Collision Demux/Contact Point Bus Creator ==
  demux in : Inport
  Bus Creator : BusCreator  Inputs=3
  Bus Creator1 : BusCreator  Inputs=3
  Bus Creator2 : BusCreator  Inputs=3
  Demux : Demux  Outputs=3
  Demux5 : Demux  Outputs=[3 3 1]
  Demux6 : Demux  Outputs=3
  bus out : Outport
  wires:
  Bus Creator1/1 -> Bus Creator2/2  "position"
  Bus Creator/1 -> Bus Creator2/1  "normal"
  Demux5/2 -> Demux6/1
  Demux5/1 -> Demux/1
  Bus Creator2/1 -> bus out/1
  Demux5/3 -> Bus Creator2/3  "penetrationdepth"
  demux in/1 -> Demux5/1
  Demux6/3 -> Bus Creator1/3  "z"
  Demux6/2 -> Bus Creator1/2  "y"
  Demux6/1 -> Bus Creator1/1  "x"
  Demux/3 -> Bus Creator/3  "z"
  Demux/2 -> Bus Creator/2  "y"
  Demux/1 -> Bus Creator/1  "x"

== system Demo_FrictionSensor_cs/Audi_A8_1/PreScan_Contact_Sensor/Tire Collision Demux/Contact Point Bus Creator1 ==
  demux in : Inport
  Bus Creator : BusCreator  Inputs=3
  Bus Creator1 : BusCreator  Inputs=3
  Bus Creator2 : BusCreator  Inputs=3
  Demux : Demux  Outputs=3
  Demux5 : Demux  Outputs=[3 3 1]
  Demux6 : Demux  Outputs=3
  bus out : Outport
  wires:
  Bus Creator1/1 -> Bus Creator2/2  "position"
  Bus Creator/1 -> Bus Creator2/1  "normal"
  Demux5/2 -> Demux6/1
  Demux5/1 -> Demux/1
  Bus Creator2/1 -> bus out/1
  Demux5/3 -> Bus Creator2/3  "penetrationdepth"
  demux in/1 -> Demux5/1
  Demux6/3 -> Bus Creator1/3  "z"
  Demux6/2 -> Bus Creator1/2  "y"
  Demux6/1 -> Bus Creator1/1  "x"
  Demux/3 -> Bus Creator/3  "z"
  Demux/2 -> Bus Creator/2  "y"
  Demux/1 -> Bus Creator/1  "x"

== system Demo_FrictionSensor_cs/Audi_A8_1/PreScan_Contact_Sensor/Tire Collision Demux/Contact Point Bus Creator2 ==
  demux in : Inport
  Bus Creator : BusCreator  Inputs=3
  Bus Creator1 : BusCreator  Inputs=3
  Bus Creator2 : BusCreator  Inputs=3
  Demux : Demux  Outputs=3
  Demux5 : Demux  Outputs=[3 3 1]
  Demux6 : Demux  Outputs=3
  bus out : Outport
  wires:
  Bus Creator1/1 -> Bus Creator2/2  "position"
  Bus Creator/1 -> Bus Creator2/1  "normal"
  Demux5/2 -> Demux6/1
  Demux5/1 -> Demux/1
  Bus Creator2/1 -> bus out/1
  Demux5/3 -> Bus Creator2/3  "penetrationdepth"
  demux in/1 -> Demux5/1
  Demux6/3 -> Bus Creator1/3  "z"
  Demux6/2 -> Bus Creator1/2  "y"
  Demux6/1 -> Bus Creator1/1  "x"
  Demux/3 -> Bus Creator/3  "z"
  Demux/2 -> Bus Creator/2  "y"
  Demux/1 -> Bus Creator/1  "x"

== system Demo_FrictionSensor_cs/Audi_A8_1/PreScan_Contact_Sensor/Tire Collision Demux/Contact Point Bus Creator3 ==
  demux in : Inport
  Bus Creator : BusCreator  Inputs=3
  Bus Creator1 : BusCreator  Inputs=3
  Bus Creator2 : BusCreator  Inputs=3
  Demux : Demux  Outputs=3
  Demux5 : Demux  Outputs=[3 3 1]
  Demux6 : Demux  Outputs=3
  bus out : Outport
  wires:
  Bus Creator1/1 -> Bus Creator2/2  "position"
  Bus Creator/1 -> Bus Creator2/1  "normal"
  Demux5/2 -> Demux6/1
  Demux5/1 -> Demux/1
  Bus Creator2/1 -> bus out/1
  Demux5/3 -> Bus Creator2/3  "penetrationdepth"
  demux in/1 -> Demux5/1
  Demux6/3 -> Bus Creator1/3  "z"
  Demux6/2 -> Bus Creator1/2  "y"
  Demux6/1 -> Bus Creator1/1  "x"
  Demux/3 -> Bus Creator/3  "z"
  Demux/2 -> Bus Creator/2  "y"
  Demux/1 -> Bus Creator/1  "x"

== system Demo_FrictionSensor_cs/Audi_A8_1/PreScan_Contact_Sensor/Tire Collision Demux1/Contact Point Bus Creator ==
  demux in : Inport
  Bus Creator : BusCreator  Inputs=3
  Bus Creator1 : BusCreator  Inputs=3
  Bus Creator2 : BusCreator  Inputs=3
  Demux : Demux  Outputs=3
  Demux5 : Demux  Outputs=[3 3 1]
  Demux6 : Demux  Outputs=3
  bus out : Outport
  wires:
  Bus Creator1/1 -> Bus Creator2/2  "position"
  Bus Creator/1 -> Bus Creator2/1  "normal"
  Demux5/2 -> Demux6/1
  Demux5/1 -> Demux/1
  Bus Creator2/1 -> bus out/1
  Demux5/3 -> Bus Creator2/3  "penetrationdepth"
  demux in/1 -> Demux5/1
  Demux6/3 -> Bus Creator1/3  "z"
  Demux6/2 -> Bus Creator1/2  "y"
  Demux6/1 -> Bus Creator1/1  "x"
  Demux/3 -> Bus Creator/3  "z"
  Demux/2 -> Bus Creator/2  "y"
  Demux/1 -> Bus Creator/1  "x"

== system Demo_FrictionSensor_cs/Audi_A8_1/PreScan_Contact_Sensor/Tire Collision Demux1/Contact Point Bus Creator1 ==
  demux in : Inport
  Bus Creator : BusCreator  Inputs=3
  Bus Creator1 : BusCreator  Inputs=3
  Bus Creator2 : BusCreator  Inputs=3
  Demux : Demux  Outputs=3
  Demux5 : Demux  Outputs=[3 3 1]
  Demux6 : Demux  Outputs=3
  bus out : Outport
  wires:
  Bus Creator1/1 -> Bus Creator2/2  "position"
  Bus Creator/1 -> Bus Creator2/1  "normal"
  Demux5/2 -> Demux6/1
  Demux5/1 -> Demux/1
  Bus Creator2/1 -> bus out/1
  Demux5/3 -> Bus Creator2/3  "penetrationdepth"
  demux in/1 -> Demux5/1
  Demux6/3 -> Bus Creator1/3  "z"
  Demux6/2 -> Bus Creator1/2  "y"
  Demux6/1 -> Bus Creator1/1  "x"
  Demux/3 -> Bus Creator/3  "z"
  Demux/2 -> Bus Creator/2  "y"
  Demux/1 -> Bus Creator/1  "x"

== system Demo_FrictionSensor_cs/Audi_A8_1/PreScan_Contact_Sensor/Tire Collision Demux1/Contact Point Bus Creator2 ==
  demux in : Inport
  Bus Creator : BusCreator  Inputs=3
  Bus Creator1 : BusCreator  Inputs=3
  Bus Creator2 : BusCreator  Inputs=3
  Demux : Demux  Outputs=3
  Demux5 : Demux  Outputs=[3 3 1]
  Demux6 : Demux  Outputs=3
  bus out : Outport
  wires:
  Bus Creator1/1 -> Bus Creator2/2  "position"
  Bus Creator/1 -> Bus Creator2/1  "normal"
  Demux5/2 -> Demux6/1
  Demux5/1 -> Demux/1
  Bus Creator2/1 -> bus out/1
  Demux5/3 -> Bus Creator2/3  "penetrationdepth"
  demux in/1 -> Demux5/1
  Demux6/3 -> Bus Creator1/3  "z"
  Demux6/2 -> Bus Creator1/2  "y"
  Demux6/1 -> Bus Creator1/1  "x"
  Demux/3 -> Bus Creator/3  "z"
  Demux/2 -> Bus Creator/2  "y"
  Demux/1 -> Bus Creator/1  "x"

== system Demo_FrictionSensor_cs/Audi_A8_1/PreScan_Contact_Sensor/Tire Collision Demux1/Contact Point Bus Creator3 ==
  demux in : Inport
  Bus Creator : BusCreator  Inputs=3
  Bus Creator1 : BusCreator  Inputs=3
  Bus Creator2 : BusCreator  Inputs=3
  Demux : Demux  Outputs=3
  Demux5 : Demux  Outputs=[3 3 1]
  Demux6 : Demux  Outputs=3
  bus out : Outport
  wires:
  Bus Creator1/1 -> Bus Creator2/2  "position"
  Bus Creator/1 -> Bus Creator2/1  "normal"
  Demux5/2 -> Demux6/1
  Demux5/1 -> Demux/1
  Bus Creator2/1 -> bus out/1
  Demux5/3 -> Bus Creator2/3  "penetrationdepth"
  demux in/1 -> Demux5/1
  Demux6/3 -> Bus Creator1/3  "z"
  Demux6/2 -> Bus Creator1/2  "y"
  Demux6/1 -> Bus Creator1/1  "x"
  Demux/3 -> Bus Creator/3  "z"
  Demux/2 -> Bus Creator/2  "y"
  Demux/1 -> Bus Creator/1  "x"

== system Demo_FrictionSensor_cs/Audi_A8_1/PreScan_Contact_Sensor/Tire Collision Demux2/Contact Point Bus Creator ==
  demux in : Inport
  Bus Creator : BusCreator  Inputs=3
  Bus Creator1 : BusCreator  Inputs=3
  Bus Creator2 : BusCreator  Inputs=3
  Demux : Demux  Outputs=3
  Demux5 : Demux  Outputs=[3 3 1]
  Demux6 : Demux  Outputs=3
  bus out : Outport
  wires:
  Bus Creator1/1 -> Bus Creator2/2  "position"
  Bus Creator/1 -> Bus Creator2/1  "normal"
  Demux5/2 -> Demux6/1
  Demux5/1 -> Demux/1
  Bus Creator2/1 -> bus out/1
  Demux5/3 -> Bus Creator2/3  "penetrationdepth"
  demux in/1 -> Demux5/1
  Demux6/3 -> Bus Creator1/3  "z"
  Demux6/2 -> Bus Creator1/2  "y"
  Demux6/1 -> Bus Creator1/1  "x"
  Demux/3 -> Bus Creator/3  "z"
  Demux/2 -> Bus Creator/2  "y"
  Demux/1 -> Bus Creator/1  "x"

== system Demo_FrictionSensor_cs/Audi_A8_1/PreScan_Contact_Sensor/Tire Collision Demux2/Contact Point Bus Creator1 ==
  demux in : Inport
  Bus Creator : BusCreator  Inputs=3
  Bus Creator1 : BusCreator  Inputs=3
  Bus Creator2 : BusCreator  Inputs=3
  Demux : Demux  Outputs=3
  Demux5 : Demux  Outputs=[3 3 1]
  Demux6 : Demux  Outputs=3
  bus out : Outport
  wires:
  Bus Creator1/1 -> Bus Creator2/2  "position"
  Bus Creator/1 -> Bus Creator2/1  "normal"
  Demux5/2 -> Demux6/1
  Demux5/1 -> Demux/1
  Bus Creator2/1 -> bus out/1
  Demux5/3 -> Bus Creator2/3  "penetrationdepth"
  demux in/1 -> Demux5/1
  Demux6/3 -> Bus Creator1/3  "z"
  Demux6/2 -> Bus Creator1/2  "y"
  Demux6/1 -> Bus Creator1/1  "x"
  Demux/3 -> Bus Creator/3  "z"
  Demux/2 -> Bus Creator/2  "y"
  Demux/1 -> Bus Creator/1  "x"

== system Demo_FrictionSensor_cs/Audi_A8_1/PreScan_Contact_Sensor/Tire Collision Demux2/Contact Point Bus Creator2 ==
  demux in : Inport
  Bus Creator : BusCreator  Inputs=3
  Bus Creator1 : BusCreator  Inputs=3
  Bus Creator2 : BusCreator  Inputs=3
  Demux : Demux  Outputs=3
  Demux5 : Demux  Outputs=[3 3 1]
  Demux6 : Demux  Outputs=3
  bus out : Outport
  wires:
  Bus Creator1/1 -> Bus Creator2/2  "position"
  Bus Creator/1 -> Bus Creator2/1  "normal"
  Demux5/2 -> Demux6/1
  Demux5/1 -> Demux/1
  Bus Creator2/1 -> bus out/1
  Demux5/3 -> Bus Creator2/3  "penetrationdepth"
  demux in/1 -> Demux5/1
  Demux6/3 -> Bus Creator1/3  "z"
  Demux6/2 -> Bus Creator1/2  "y"
  Demux6/1 -> Bus Creator1/1  "x"
  Demux/3 -> Bus Creator/3  "z"
  Demux/2 -> Bus Creator/2  "y"
  Demux/1 -> Bus Creator/1  "x"

== system Demo_FrictionSensor_cs/Audi_A8_1/PreScan_Contact_Sensor/Tire Collision Demux2/Contact Point Bus Creator3 ==
  demux in : Inport
  Bus Creator : BusCreator  Inputs=3
  Bus Creator1 : BusCreator  Inputs=3
  Bus Creator2 : BusCreator  Inputs=3
  Demux : Demux  Outputs=3
  Demux5 : Demux  Outputs=[3 3 1]
  Demux6 : Demux  Outputs=3
  bus out : Outport
  wires:
  Bus Creator1/1 -> Bus Creator2/2  "position"
  Bus Creator/1 -> Bus Creator2/1  "normal"
  Demux5/2 -> Demux6/1
  Demux5/1 -> Demux/1
  Bus Creator2/1 -> bus out/1
  Demux5/3 -> Bus Creator2/3  "penetrationdepth"
  demux in/1 -> Demux5/1
  Demux6/3 -> Bus Creator1/3  "z"
  Demux6/2 -> Bus Creator1/2  "y"
  Demux6/1 -> Bus Creator1/1  "x"
  Demux/3 -> Bus Creator/3  "z"
  Demux/2 -> Bus Creator/2  "y"
  Demux/1 -> Bus Creator/1  "x"

== system Demo_FrictionSensor_cs/Audi_A8_1/PreScan_Contact_Sensor/Tire Collision Demux3/Contact Point Bus Creator ==
  demux in : Inport
  Bus Creator : BusCreator  Inputs=3
  Bus Creator1 : BusCreator  Inputs=3
  Bus Creator2 : BusCreator  Inputs=3
  Demux : Demux  Outputs=3
  Demux5 : Demux  Outputs=[3 3 1]
  Demux6 : Demux  Outputs=3
  bus out : Outport
  wires:
  Bus Creator1/1 -> Bus Creator2/2  "position"
  Bus Creator/1 -> Bus Creator2/1  "normal"
  Demux5/2 -> Demux6/1
  Demux5/1 -> Demux/1
  Bus Creator2/1 -> bus out/1
  Demux5/3 -> Bus Creator2/3  "penetrationdepth"
  demux in/1 -> Demux5/1
  Demux6/3 -> Bus Creator1/3  "z"
  Demux6/2 -> Bus Creator1/2  "y"
  Demux6/1 -> Bus Creator1/1  "x"
  Demux/3 -> Bus Creator/3  "z"
  Demux/2 -> Bus Creator/2  "y"
  Demux/1 -> Bus Creator/1  "x"

== system Demo_FrictionSensor_cs/Audi_A8_1/PreScan_Contact_Sensor/Tire Collision Demux3/Contact Point Bus Creator1 ==
  demux in : Inport
  Bus Creator : BusCreator  Inputs=3
  Bus Creator1 : BusCreator  Inputs=3
  Bus Creator2 : BusCreator  Inputs=3
  Demux : Demux  Outputs=3
  Demux5 : Demux  Outputs=[3 3 1]
  Demux6 : Demux  Outputs=3
  bus out : Outport
  wires:
  Bus Creator1/1 -> Bus Creator2/2  "position"
  Bus Creator/1 -> Bus Creator2/1  "normal"
  Demux5/2 -> Demux6/1
  Demux5/1 -> Demux/1
  Bus Creator2/1 -> bus out/1
  Demux5/3 -> Bus Creator2/3  "penetrationdepth"
  demux in/1 -> Demux5/1
  Demux6/3 -> Bus Creator1/3  "z"
  Demux6/2 -> Bus Creator1/2  "y"
  Demux6/1 -> Bus Creator1/1  "x"
  Demux/3 -> Bus Creator/3  "z"
  Demux/2 -> Bus Creator/2  "y"
  Demux/1 -> Bus Creator/1  "x"

== system Demo_FrictionSensor_cs/Audi_A8_1/PreScan_Contact_Sensor/Tire Collision Demux3/Contact Point Bus Creator2 ==
  demux in : Inport
  Bus Creator : BusCreator  Inputs=3
  Bus Creator1 : BusCreator  Inputs=3
  Bus Creator2 : BusCreator  Inputs=3
  Demux : Demux  Outputs=3
  Demux5 : Demux  Outputs=[3 3 1]
  Demux6 : Demux  Outputs=3
  bus out : Outport
  wires:
  Bus Creator1/1 -> Bus Creator2/2  "position"
  Bus Creator/1 -> Bus Creator2/1  "normal"
  Demux5/2 -> Demux6/1
  Demux5/1 -> Demux/1
  Bus Creator2/1 -> bus out/1
  Demux5/3 -> Bus Creator2/3  "penetrationdepth"
  demux in/1 -> Demux5/1
  Demux6/3 -> Bus Creator1/3  "z"
  Demux6/2 -> Bus Creator1/2  "y"
  Demux6/1 -> Bus Creator1/1  "x"
  Demux/3 -> Bus Creator/3  "z"
  Demux/2 -> Bus Creator/2  "y"
  Demux/1 -> Bus Creator/1  "x"

== system Demo_FrictionSensor_cs/Audi_A8_1/PreScan_Contact_Sensor/Tire Collision Demux3/Contact Point Bus Creator3 ==
  demux in : Inport
  Bus Creator : BusCreator  Inputs=3
  Bus Creator1 : BusCreator  Inputs=3
  Bus Creator2 : BusCreator  Inputs=3
  Demux : Demux  Outputs=3
  Demux5 : Demux  Outputs=[3 3 1]
  Demux6 : Demux  Outputs=3
  bus out : Outport
  wires:
  Bus Creator1/1 -> Bus Creator2/2  "position"
  Bus Creator/1 -> Bus Creator2/1  "normal"
  Demux5/2 -> Demux6/1
  Demux5/1 -> Demux/1
  Bus Creator2/1 -> bus out/1
  Demux5/3 -> Bus Creator2/3  "penetrationdepth"
  demux in/1 -> Demux5/1
  Demux6/3 -> Bus Creator1/3  "z"
  Demux6/2 -> Bus Creator1/2  "y"
  Demux6/1 -> Bus Creator1/1  "x"
  Demux/3 -> Bus Creator/3  "z"
  Demux/2 -> Bus Creator/2  "y"
  Demux/1 -> Bus Creator/1  "x"

== system Demo_FrictionSensor_cs/Audi_A8_1/PreScan_Contact_Sensor/Vehicle Local to World/state2FullState ==
  note: AnglesBODY
      | wrtVEH
  note: AnglesVEHICLE
      | wrtGLOB
  note: AnglesBODY
      | wrt GLOB
  note: mode: Dynamics
      | VelVEHICLE
      | wrt VEH
  note: mode: Positioning
      | VelVEHICLE
      | wrt INI
  note: Angles
      | wrtINI
  note: wrt GLOB
  dx,dy,dz [m/s] R,P,Y  [rad] : Inport
  ini VEHpos wrt GLOB axis system  [m] : Inport  Port=2
  iniBODY Angles wrt VEH axis system [deg] : Inport  Port=3
  iniVEH Angles wrt GLOB axis system [deg] : Inport  Port=4
  Degrees to Radians : simulink_extras/Transformations/Degrees to Radians  SystemSampleTime=-1
  Degrees to Radians1 : simulink_extras/Transformations/Degrees to Radians  SystemSampleTime=-1
  Demux1 : Demux  Outputs=[3 3 3]
  Demux2 : Demux  Outputs=[2 1]
  Demux3 : Demux  Outputs=2
  Mux : Mux  Inputs=[3 3]
  Sum : Sum  Inputs=|++
  Sum1 : Sum
  Sum2 : Sum
  Sum3 : Sum
  Terminator : Terminator
  Transformation_BODY2GLOBAL1 : Subsystem
  limit roll : Subsystem
  mux2 : Mux  Inputs=3
  mux3 : Mux  Inputs=3
  pitch_vehicle : Constant  Value=0
  roll_vehicle : Constant  Value=0
  yaw_body : Constant  Value=0
  State : Outport
  wires:
  Demux1/2 -> Terminator/1
  limit roll/1(RPYcor) -> Mux/2  "AnglesBODY wrt  GLOB"
  Mux/1 -> State/1
  iniVEH Angles wrt GLOB axis system [deg]/1 -> Degrees to Radians/1
  iniBODY Angles wrt VEH axis system [deg]/1 -> Degrees to Radians1/1
  Sum/1 -> limit roll/1(RPY)
  roll_vehicle/1 -> mux3/1  "roll"
  pitch_vehicle/1 -> mux3/2  "pitch"
  mux2/1 -> Sum1/1
  yaw_body/1 -> mux2/3  "yaw"
  mux3/1 -> Sum2/1
  Sum2/1 -> Sum/2
  dx,dy,dz [m/s] R,P,Y  [rad]/1 -> Demux1/1
  Demux1/1 -> Transformation_BODY2GLOBAL1/1(POSvector_BODY_[m])
  Sum1/1 -> Sum/1
  Transformation_BODY2GLOBAL1/1(POSvector_GLOBAL_[m]) -> Sum3/1
  Sum3/1 -> Mux/1  "PosVEH wrt  GLOB"
  Demux2/2 -> mux3/3  "yaw"
  Demux2/1 -> Demux3/1
  Demux1/3 -> Demux2/1
  Demux3/1 -> mux2/1  "roll"
  Degrees to Radians1/1 -> Sum1/2
  Degrees to Radians/1 -> Transformation_BODY2GLOBAL1/2(angles_BODYwrtGLOB_[rad]), Sum2/2
  ini VEHpos wrt GLOB axis system  [m]/1 -> Sum3/2
  Demux3/2 -> mux2/2  "pitch"
